simulink model "truck_van_damme"  (R2022a)
settings: Solver=VariableStepAuto  StartTime=0.0  StopTime=100  MaxStep=0.01  RelTol=1e-3
settings Model: Creator=hansae  LastModifiedBy=hansae
settings ModelReferenceCC: EnableRefExpFcnMdlSchedulingChecks=off
settings RTWCC: Description=Generic Real-Time Target

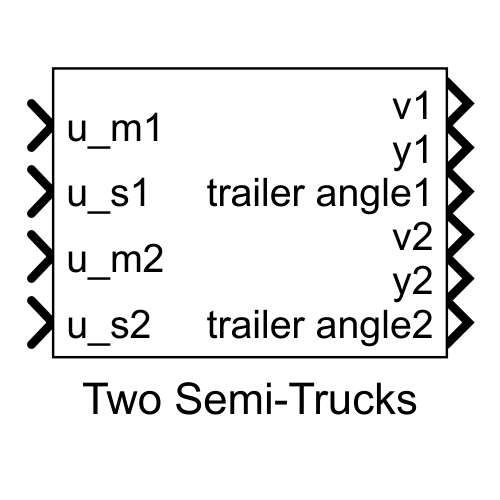
[thumbnail: Simulink's stored preview of the top-level diagram]
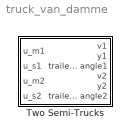
== system truck_van_damme ==
  Two Semi-Trucks : Subsystem

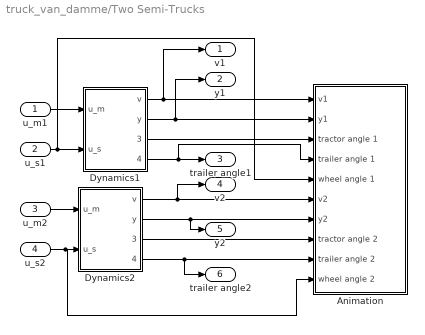
== system truck_van_damme/Two Semi-Trucks ==
  u_m1 : Inport
  u_s1 : Inport  Port=2
  u_m2 : Inport  Port=3
  u_s2 : Inport  Port=4
  Animation : Subsystem
  Dynamics1 : Subsystem  ClipboardFcn=parameters_truck.m
  Dynamics2 : Subsystem  ClipboardFcn=parameters_truck.m
  v1 : Outport
  y1 : Outport  Port=2
  trailer angle1 : Outport  Port=3
  v2 : Outport  Port=4
  y2 : Outport  Port=5
  trailer angle2 : Outport  Port=6
  wires:
  Dynamics1/2(y) -> y1/1, Animation/2(y1)
  u_s1/1 -> Animation/5(wheel angle 1), Dynamics1/2(u_s)
  u_m1/1 -> Dynamics1/1(u_m)
  Dynamics1/3(tractor angle) -> Animation/3(tractor angle 1)
  Dynamics1/4(trailer angle) -> Animation/4(trailer angle 1), trailer angle1/1
  u_s2/1 -> Animation/10(wheel angle 2), Dynamics2/2(u_s)
  Dynamics2/3(tractor angle) -> Animation/8(tractor angle 2)
  Dynamics2/4(trailer angle) -> trailer angle2/1, Animation/9(trailer angle 2)
  Dynamics1/1(v) -> v1/1, Animation/1(v1)
  Dynamics2/1(v) -> v2/1, Animation/6(v2)
  Dynamics2/2(y) -> Animation/7(y2), y2/1
  u_m2/1 -> Dynamics2/1(u_m)

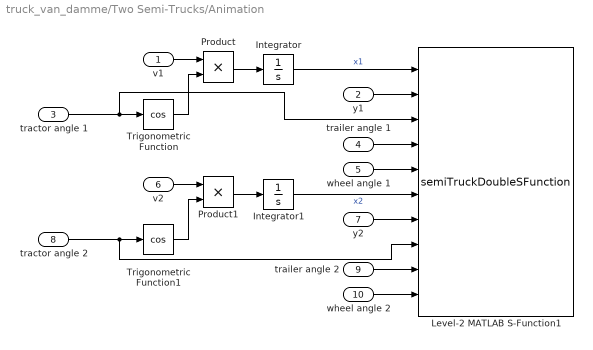
== system truck_van_damme/Two Semi-Trucks/Animation ==
  v1 : Inport
  y1 : Inport  Port=2
  tractor angle 1 : Inport  Port=3
  trailer angle 1 : Inport  Port=4
  wheel angle 1 : Inport  Port=5
  v2 : Inport  Port=6
  y2 : Inport  Port=7
  tractor angle 2 : Inport  Port=8
  trailer angle 2 : Inport  Port=9
  wheel angle 2 : Inport  Port=10
  Integrator : Integrator
  Integrator1 : Integrator
  Level-2 MATLAB S-Function1 : M-S-Function  FunctionName=semiTruckDoubleSFunction
  Product : Product
  Product1 : Product
  Trigonometric Function : Trigonometry  Operator=cos
  Trigonometric Function1 : Trigonometry  Operator=cos
  wires:
  Product/1 -> Integrator/1
  Trigonometric Function/1 -> Product/2
  v1/1 -> Product/1
  y1/1 -> Level-2 MATLAB S-Function1/2
  Integrator/1 -> Level-2 MATLAB S-Function1/1  "x1"
  tractor angle 1/1 -> Trigonometric Function/1, Level-2 MATLAB S-Function1/3
  wheel angle 1/1 -> Level-2 MATLAB S-Function1/5
  trailer angle 1/1 -> Level-2 MATLAB S-Function1/4
  Product1/1 -> Integrator1/1
  Trigonometric Function1/1 -> Product1/2
  v2/1 -> Product1/1
  tractor angle 2/1 -> Level-2 MATLAB S-Function1/8, Trigonometric Function1/1
  Integrator1/1 -> Level-2 MATLAB S-Function1/6  "x2"
  y2/1 -> Level-2 MATLAB S-Function1/7
  trailer angle 2/1 -> Level-2 MATLAB S-Function1/9
  wheel angle 2/1 -> Level-2 MATLAB S-Function1/10

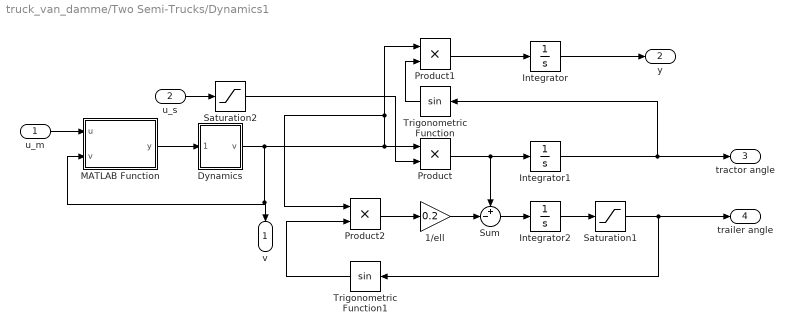
== system truck_van_damme/Two Semi-Trucks/Dynamics1 ==
  u_m : Inport
  u_s : Inport  Port=2
  1/ell : Gain  Gain=0.2
  Dynamics : Subsystem  ClipboardFcn=parameters_truck.m
  Integrator : Integrator  InitialCondition=1.25
  Integrator1 : Integrator
  Integrator2 : Integrator
  MATLAB Function : MATLAB Function  TreatAsAtomicUnit=on
  Product : Product
  Product1 : Product
  Product2 : Product
  Saturation1 : Saturate  UpperLimit=pi/2  LowerLimit=-pi/2
  Saturation2 : Saturate  UpperLimit=pi/4  LowerLimit=-pi/4
  Sum : Sum  Inputs=+-|
  Trigonometric Function : Trigonometry
  Trigonometric Function1 : Trigonometry
  v : Outport
  y : Outport  Port=2
  tractor angle : Outport  Port=3
  trailer angle : Outport  Port=4
  wires:
  Integrator/1 -> y/1
  Product/1 -> Integrator1/1, Sum/1
  Product1/1 -> Integrator/1
  Trigonometric Function/1 -> Product1/2
  Integrator2/1 -> Saturation1/1
  Trigonometric Function1/1 -> Product2/2
  Product2/1 -> 1/ell/1
  Sum/1 -> Integrator2/1
  1/ell/1 -> Sum/2
  Saturation2/1 -> Product/2
  Integrator1/1 -> tractor angle/1, Trigonometric Function/1
  Saturation1/1 -> trailer angle/1, Trigonometric Function1/1
  u_s/1 -> Saturation2/1
  MATLAB Function/1(y) -> Dynamics/1(u_m)
  u_m/1 -> MATLAB Function/1(u)
  Dynamics/1(v) -> v/1, MATLAB Function/2(v), Product2/1, Product1/1, Product/1

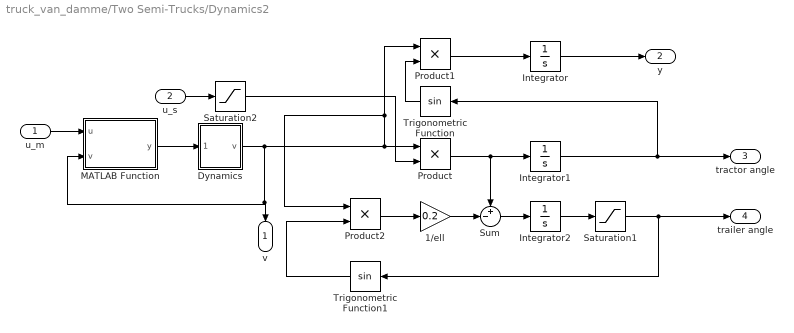
== system truck_van_damme/Two Semi-Trucks/Dynamics2 ==
  u_m : Inport
  u_s : Inport  Port=2
  1/ell : Gain  Gain=0.2
  Dynamics : Subsystem  ClipboardFcn=parameters_truck.m
  Integrator : Integrator  InitialCondition=-1.25
  Integrator1 : Integrator
  Integrator2 : Integrator
  MATLAB Function : MATLAB Function  TreatAsAtomicUnit=on
  Product : Product
  Product1 : Product
  Product2 : Product
  Saturation1 : Saturate  UpperLimit=pi/2  LowerLimit=-pi/2
  Saturation2 : Saturate  UpperLimit=pi/4  LowerLimit=-pi/4
  Sum : Sum  Inputs=+-|
  Trigonometric Function : Trigonometry
  Trigonometric Function1 : Trigonometry
  v : Outport
  y : Outport  Port=2
  tractor angle : Outport  Port=3
  trailer angle : Outport  Port=4
  wires:
  Integrator/1 -> y/1
  Product/1 -> Integrator1/1, Sum/1
  Product1/1 -> Integrator/1
  Trigonometric Function/1 -> Product1/2
  Integrator2/1 -> Saturation1/1
  Trigonometric Function1/1 -> Product2/2
  Product2/1 -> 1/ell/1
  Sum/1 -> Integrator2/1
  1/ell/1 -> Sum/2
  Saturation2/1 -> Product/2
  Integrator1/1 -> tractor angle/1, Trigonometric Function/1
  Saturation1/1 -> trailer angle/1, Trigonometric Function1/1
  u_s/1 -> Saturation2/1
  MATLAB Function/1(y) -> Dynamics/1(u_m)
  u_m/1 -> MATLAB Function/1(u)
  Dynamics/1(v) -> v/1, MATLAB Function/2(v), Product2/1, Product1/1, Product/1

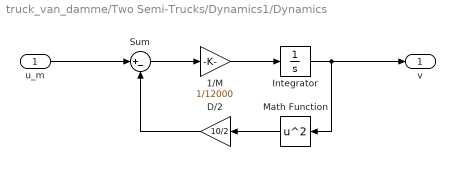
== system truck_van_damme/Two Semi-Trucks/Dynamics1/Dynamics ==
  u_m : Inport
  1/M : Gain  Gain=1/12000
  D/2 : Gain  Gain=10/2
  Integrator : Integrator
  Math Function : Math  Operator=square
  Sum : Sum  Inputs=|+-
  v : Outport
  wires:
  Integrator/1 -> v/1, Math Function/1
  Sum/1 -> 1/M/1
  u_m/1 -> Sum/1
  1/M/1 -> Integrator/1
  D/2/1 -> Sum/2
  Math Function/1 -> D/2/1

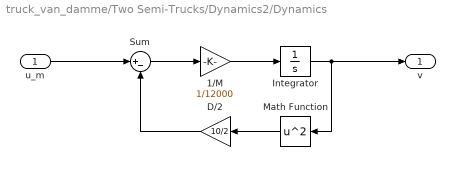
== system truck_van_damme/Two Semi-Trucks/Dynamics2/Dynamics ==
  u_m : Inport
  1/M : Gain  Gain=1/12000
  D/2 : Gain  Gain=10/2
  Integrator : Integrator
  Math Function : Math  Operator=square
  Sum : Sum  Inputs=|+-
  v : Outport
  wires:
  Integrator/1 -> v/1, Math Function/1
  Sum/1 -> 1/M/1
  u_m/1 -> Sum/1
  1/M/1 -> Integrator/1
  D/2/1 -> Sum/2
  Math Function/1 -> D/2/1

== matlab function truck_van_damme/Two Semi-Trucks/Dynamics2/MATLAB Function ==
  data: u input; y output; v input
function y = saturation(u,v)
    Pmax = 400000;
    epsilon = 0.1;
    
    sat = Pmax/sqrt(v^2+epsilon);
    y = max(min(u,sat),-sat);

== matlab function truck_van_damme/Two Semi-Trucks/Dynamics1/MATLAB Function ==
  data: u input; y output; v input
function y = saturation(u,v)
    Pmax = 400000;
    epsilon = 0.1;
    
    sat = Pmax/sqrt(v^2+epsilon);
    y = max(min(u,sat),-sat);
